simulink model "fan_model"  (R2024b)
settings: Solver=FixedStepDiscrete  StartTime=0.0  StopTime=100  FixedStep=1e-4  RelTol=1e-3
values from neighbouring files (symbols this model uses):
  a = 0.0    [data.sldd]
  J_f = 0.0    [data.sldd]
  J_m = 0.0    [data.sldd]
  Speed_max = 0.0    [data.sldd]
  T0 = 0.0    [data.sldd]
  Torque_max = 0.0    [data.sldd]
undefined symbols (not defined in the file or in its folder): DiscIntNeverNeededParam
settings Model: DataDictionary=data.sldd  Creator=SESA504213  LastModifiedBy=SESA504213

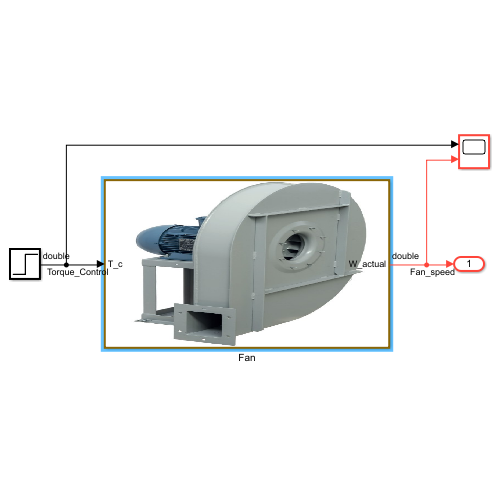
[thumbnail: Simulink's stored preview of the top-level diagram]
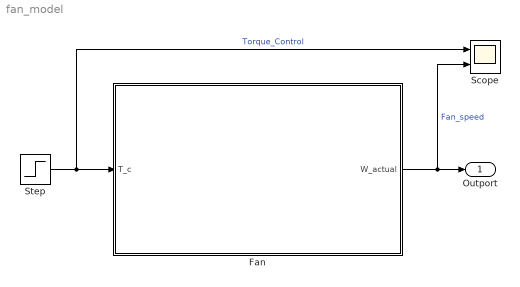
== system fan_model ==
  Fan : Subsystem
      mask Display: image('FanwithMotor.jpg');
  Scope : Scope  NumInputPorts=2
  Step : Step  After=13.12  SampleTime=0
  Outport : Outport
  wires:
  Fan/1(W_actual) -> Outport/1, Scope/2  "Fan_speed"
  Step/1 -> Scope/1, Fan/1(T_c)  "Torque_Control"

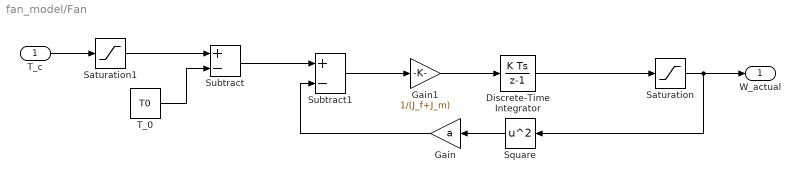
== system fan_model/Fan ==
  T_c : Inport
  Discrete-Time Integrator : DiscreteIntegrator  SampleTime=-1  ICPrevOutput=DiscIntNeverNeededParam  ICPrevScaledInput=DiscIntNeverNeededParam
  Gain : Gain  Gain=a
  Gain1 : Gain  Gain=1/(J_f+J_m)
  Saturation : Saturate  UpperLimit=Speed_max  LowerLimit=-Speed_max
  Saturation1 : Saturate  UpperLimit=Torque_max  LowerLimit=-Torque_max
  Square : Math  Operator=square
  Subtract : Sum  Inputs=+-
  Subtract1 : Sum  Inputs=+-
  T_0 : Constant  Value=T0
  W_actual : Outport
  wires:
  Gain1/1 -> Discrete-Time Integrator/1
  Square/1 -> Gain/1
  T_c/1 -> Saturation1/1
  T_0/1 -> Subtract/2
  Subtract1/1 -> Gain1/1
  Discrete-Time Integrator/1 -> Saturation/1
  Subtract/1 -> Subtract1/1
  Gain/1 -> Subtract1/2
  Saturation/1 -> Square/1, W_actual/1
  Saturation1/1 -> Subtract/1
